simulink model "model"  (R2015a)
settings: Solver=ode45  StartTime=0.0  StopTime=16  RelTol=1e-3
values from neighbouring files (symbols this model uses):
  flc = addrule(flc,rule)    [createFLC.m]
libraries: checkpacklib x1, fuzblock x1
settings Model: Creator=Raft  LastModifiedBy=Raft

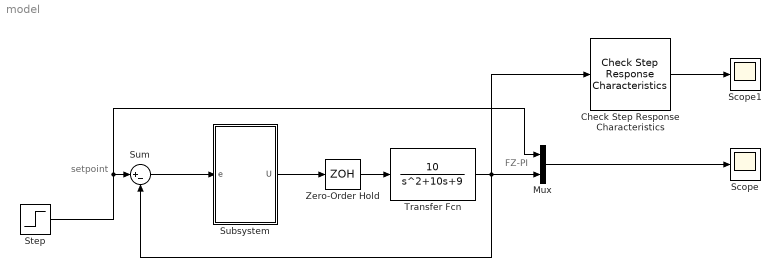
== system model ==
  note: FZ-PI
  note: setpoint
  Check Step Response Characteristics : checkpacklib/Check Step Response  Characteristics  InstantiateOnLoad=on  enabled=on  stopWhenAssertionFail=off  export=on  ViewDlgPos=[100 200 510 390]  OpenViewOnLoad=off  LaunchViewOnOpen=off  TimeUnits=seconds  EnableStepResponseBound=on  InitialValue=0  FinalValue=1  StepTime=10  RiseTime=0.6  PercentRise=90  SettlingTime=3  PercentSettling=7  PercentOvershoot=7  PercentUndershoot=100  ZeroCross=off
  Mux : Mux  Inputs=2
  Scope : Scope
      settings: TickLabels=on  ShowLegends=on  YMin=0  YMax=65  SaveName=sysOutboth
  Scope1 : Scope
  Step : Step  Time=0  SampleTime=0
  Subsystem : Subsystem
  Sum : Sum  Inputs=|+-
  Transfer Fcn : TransferFcn  Numerator=[10]  Denominator=[1 10 9]
  Zero-Order Hold : ZeroOrderHold  SampleTime=0.01
  wires:
  Sum/1 -> Subsystem/1(e)
  Step/1 -> Mux/1, Sum/1
  Subsystem/1(U) -> Zero-Order Hold/1
  Zero-Order Hold/1 -> Transfer Fcn/1
  Transfer Fcn/1 -> Check Step Response Characteristics/1, Sum/2, Mux/2
  Mux/1 -> Scope/1
  Check Step Response Characteristics/1 -> Scope1/1

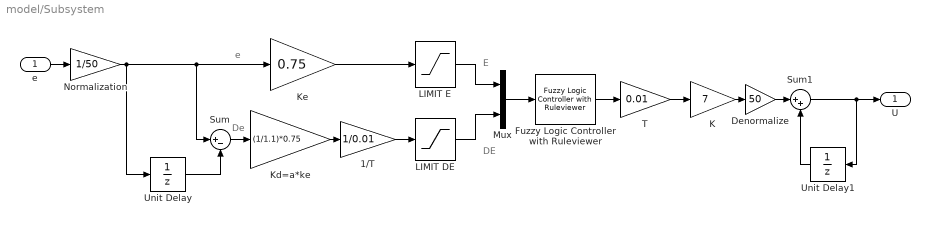
== system model/Subsystem ==
  note: DE
  note: E
  note: De
  note: e
  e : Inport
  1/T : Gain  Gain=1/0.01
  Denormalize : Gain  Gain=50
  Fuzzy Logic Controller with Ruleviewer : fuzblock/Fuzzy Logic  Controller  with Ruleviewer  fismatrix=[flc]  Ts=0.8
  K : Gain  Gain=7
  Kd=a*ke : Gain  Gain=(1/1.1)*0.75
  Ke : Gain  Gain=0.75
  LIMIT DE : Saturate  UpperLimit=1  LowerLimit=-1
  LIMIT E : Saturate  UpperLimit=1  LowerLimit=-1
  Mux : Mux  Inputs=2
  Normalization : Gain  Gain=1/50
  Sum : Sum  Inputs=|+-
  Sum1 : Sum  Inputs=|++
  T : Gain  Gain=0.01
  Unit Delay : UnitDelay  SampleTime=0.01
  Unit Delay1 : UnitDelay  SampleTime=0.01
  U : Outport
  wires:
  1/T/1 -> LIMIT DE/1
  Mux/1 -> Fuzzy Logic Controller with Ruleviewer/1
  Denormalize/1 -> Sum1/1
  LIMIT DE/1 -> Mux/2
  LIMIT E/1 -> Mux/1
  Sum1/1 -> Unit Delay1/1, U/1
  Unit Delay1/1 -> Sum1/2
  T/1 -> K/1
  Fuzzy Logic Controller with Ruleviewer/1 -> T/1
  Unit Delay/1 -> Sum/2
  Sum/1 -> Kd=a*ke/1
  Normalization/1 -> Unit Delay/1, Sum/1, Ke/1
  Ke/1 -> LIMIT E/1
  Kd=a*ke/1 -> 1/T/1
  e/1 -> Normalization/1
  K/1 -> Denormalize/1
